simulink model "Cooling_System"  (R2019b)
settings: Solver=VariableStepAuto  StartTime=0.0  StopTime=3600  RelTol=1e-3
libraries: fl_lib x170, nesl_utility x49
(part 2 of 2)

== system Cooling_System/segment/Cell conductance23 ==
  Air-Iron Conductance : fl_lib/Thermal/Thermal Elements/Conductive Heat Transfer  area=0.014 m^2  thickness=2 mm  th_cond=0.0257 W/(m*K)  T_specify=off  T_priority=None  T=0 K  T_nominal_specify=off  T_nominal_unit=K  T_nominal_value=1  Q_specify=off  Q_priority=None  Q=0 W  Q_nominal_specify=off  Q_nominal_unit=W  Q_nominal_value=1
      settings: SourceProductName=Simscape
  Atmosphere Temperature : fl_lib/Thermal/Thermal Sources/Temperature Source  temperature=300 K
      settings: SourceProductName=Simscape
  Jules Power Losses : fl_lib/Thermal/Thermal Sources/Controlled Heat Flow Rate Source
      settings: SourceProductName=Simscape
  PS-Simulink Converter : nesl_utility/PS-Simulink Converter  PhysicalDomain=network_engine_domain  SubClassName=ps_output  LeftPortType=input  RightPortType=output  PseudoPeriodic=off  Frequencies=[]  Unit=1  AffineConversion=off
  Simulink-PS Converter : nesl_utility/Simulink-PS Converter  PhysicalDomain=network_engine_domain  SubClassName=ps_input  LeftPortType=input  RightPortType=output  PseudoPeriodic=off  Frequencies=[]  NoiseDistribution=none  NoiseParameters=[]  Unit=W  AffineConversion=off  FilteringAndDerivatives=zero  SimscapeFilterOrder=1  InputFilterTimeConstant=.001  UdotUserProvided=[]
  Stator Iron Thermal Mass : fl_lib/Thermal/Thermal Elements/Thermal Mass  mass=0.3 kg  sp_heat=460 J/kg/K  T_specify=off  T_priority=High  T=300 K  T_nominal_specify=off  T_nominal_unit=K  T_nominal_value=1  Q_specify=off  Q_priority=None  Q=0 W  Q_nominal_specify=off  Q_nominal_unit=W  Q_nominal_value=1
  Temperature Sensor : fl_lib/Thermal/Thermal Sensors/Temperature Sensor
  Thermal Reference : fl_lib/Thermal/Thermal Elements/Thermal Reference
  Thermal Resistance : fl_lib/Thermal/Thermal Elements/Thermal Resistance  resistance=1/(1.006*1.202*0.028*50.4/60*1000) K/W  T_specify=off  T_priority=None  T=0 K  T_nominal_specify=off  T_nominal_unit=K  T_nominal_value=1  Q_specify=off  Q_priority=None  Q=0 W  Q_nominal_specify=off  Q_nominal_unit=W  Q_nominal_value=1
      settings: SourceProductName=Simscape  SourceProductBaseCode=SS
  temp_Cell_A : PMIOPort  Side=Left
  temp_Cell_B : PMIOPort  Port=2  Side=Right
  tag scope: temp_cell_23=global
  wires:
  [Q_cell] -> Simulink-PS Converter/1
  PS-Simulink Converter/1 -> [temp_cell_23]
  connections:
  Jules Power Losses/LConn1 -- temp_Cell_A/RConn1 -- Temperature Sensor/RConn1 -- Stator Iron Thermal Mass/LConn1 -- Air-Iron Conductance/LConn1
  Air-Iron Conductance/RConn1 -- Thermal Resistance/LConn1 -- temp_Cell_B/RConn1 -- Temperature Sensor/LConn1
  Atmosphere Temperature/LConn1 -- Thermal Resistance/RConn1
  Jules Power Losses/RConn1 -- Simulink-PS Converter/RConn1
  PS-Simulink Converter/LConn1 -- Temperature Sensor/RConn2
  Thermal Reference/LConn1 -- Jules Power Losses/RConn2

== system Cooling_System/segment/Cell conductance24 ==
  Air-Iron Conductance : fl_lib/Thermal/Thermal Elements/Conductive Heat Transfer  area=0.014 m^2  thickness=2 mm  th_cond=0.0257 W/(m*K)  T_specify=off  T_priority=None  T=0 K  T_nominal_specify=off  T_nominal_unit=K  T_nominal_value=1  Q_specify=off  Q_priority=None  Q=0 W  Q_nominal_specify=off  Q_nominal_unit=W  Q_nominal_value=1
      settings: SourceProductName=Simscape
  Atmosphere Temperature : fl_lib/Thermal/Thermal Sources/Temperature Source  temperature=300 K
      settings: SourceProductName=Simscape
  Jules Power Losses : fl_lib/Thermal/Thermal Sources/Controlled Heat Flow Rate Source
      settings: SourceProductName=Simscape
  PS-Simulink Converter : nesl_utility/PS-Simulink Converter  PhysicalDomain=network_engine_domain  SubClassName=ps_output  LeftPortType=input  RightPortType=output  PseudoPeriodic=off  Frequencies=[]  Unit=1  AffineConversion=off
  Simulink-PS Converter : nesl_utility/Simulink-PS Converter  PhysicalDomain=network_engine_domain  SubClassName=ps_input  LeftPortType=input  RightPortType=output  PseudoPeriodic=off  Frequencies=[]  NoiseDistribution=none  NoiseParameters=[]  Unit=W  AffineConversion=off  FilteringAndDerivatives=zero  SimscapeFilterOrder=1  InputFilterTimeConstant=.001  UdotUserProvided=[]
  Stator Iron Thermal Mass : fl_lib/Thermal/Thermal Elements/Thermal Mass  mass=0.3 kg  sp_heat=460 J/kg/K  T_specify=off  T_priority=High  T=300 K  T_nominal_specify=off  T_nominal_unit=K  T_nominal_value=1  Q_specify=off  Q_priority=None  Q=0 W  Q_nominal_specify=off  Q_nominal_unit=W  Q_nominal_value=1
  Temperature Sensor : fl_lib/Thermal/Thermal Sensors/Temperature Sensor
  Thermal Reference : fl_lib/Thermal/Thermal Elements/Thermal Reference
  Thermal Resistance : fl_lib/Thermal/Thermal Elements/Thermal Resistance  resistance=1/(1.006*1.202*0.028*50.4/60*1000) K/W  T_specify=off  T_priority=None  T=0 K  T_nominal_specify=off  T_nominal_unit=K  T_nominal_value=1  Q_specify=off  Q_priority=None  Q=0 W  Q_nominal_specify=off  Q_nominal_unit=W  Q_nominal_value=1
      settings: SourceProductName=Simscape  SourceProductBaseCode=SS
  temp_Cell_A : PMIOPort  Side=Left
  temp_Cell_B : PMIOPort  Port=2  Side=Right
  tag scope: temp_cell_24=global
  wires:
  [Q_cell] -> Simulink-PS Converter/1
  PS-Simulink Converter/1 -> [temp_cell_24]
  connections:
  Jules Power Losses/LConn1 -- temp_Cell_A/RConn1 -- Temperature Sensor/RConn1 -- Stator Iron Thermal Mass/LConn1 -- Air-Iron Conductance/LConn1
  Air-Iron Conductance/RConn1 -- Thermal Resistance/LConn1 -- temp_Cell_B/RConn1 -- Temperature Sensor/LConn1
  Atmosphere Temperature/LConn1 -- Thermal Resistance/RConn1
  Jules Power Losses/RConn1 -- Simulink-PS Converter/RConn1
  PS-Simulink Converter/LConn1 -- Temperature Sensor/RConn2
  Thermal Reference/LConn1 -- Jules Power Losses/RConn2

== system Cooling_System/segment/Cell conductance3 ==
  Air-Iron Conductance : fl_lib/Thermal/Thermal Elements/Conductive Heat Transfer  area=0.014 m^2  thickness=2 mm  th_cond=0.0257 W/(m*K)  T_specify=off  T_priority=None  T=0 K  T_nominal_specify=off  T_nominal_unit=K  T_nominal_value=1  Q_specify=off  Q_priority=None  Q=0 W  Q_nominal_specify=off  Q_nominal_unit=W  Q_nominal_value=1
      settings: SourceProductName=Simscape
  Atmosphere Temperature : fl_lib/Thermal/Thermal Sources/Temperature Source  temperature=300 K
      settings: SourceProductName=Simscape
  Jules Power Losses : fl_lib/Thermal/Thermal Sources/Controlled Heat Flow Rate Source
      settings: SourceProductName=Simscape
  PS-Simulink Converter : nesl_utility/PS-Simulink Converter  PhysicalDomain=network_engine_domain  SubClassName=ps_output  LeftPortType=input  RightPortType=output  PseudoPeriodic=off  Frequencies=[]  Unit=1  AffineConversion=off
  Simulink-PS Converter : nesl_utility/Simulink-PS Converter  PhysicalDomain=network_engine_domain  SubClassName=ps_input  LeftPortType=input  RightPortType=output  PseudoPeriodic=off  Frequencies=[]  NoiseDistribution=none  NoiseParameters=[]  Unit=W  AffineConversion=off  FilteringAndDerivatives=zero  SimscapeFilterOrder=1  InputFilterTimeConstant=.001  UdotUserProvided=[]
  Stator Iron Thermal Mass : fl_lib/Thermal/Thermal Elements/Thermal Mass  mass=0.3 kg  sp_heat=460 J/kg/K  T_specify=off  T_priority=High  T=300 K  T_nominal_specify=off  T_nominal_unit=K  T_nominal_value=1  Q_specify=off  Q_priority=None  Q=0 W  Q_nominal_specify=off  Q_nominal_unit=W  Q_nominal_value=1
  Temperature Sensor : fl_lib/Thermal/Thermal Sensors/Temperature Sensor
  Thermal Reference : fl_lib/Thermal/Thermal Elements/Thermal Reference
  Thermal Resistance : fl_lib/Thermal/Thermal Elements/Thermal Resistance  resistance=1/(1.006*1.202*0.028*50.4/60*1000) K/W  T_specify=off  T_priority=None  T=0 K  T_nominal_specify=off  T_nominal_unit=K  T_nominal_value=1  Q_specify=off  Q_priority=None  Q=0 W  Q_nominal_specify=off  Q_nominal_unit=W  Q_nominal_value=1
      settings: SourceProductName=Simscape  SourceProductBaseCode=SS
  temp_Cell_A : PMIOPort  Side=Left
  temp_Cell_B : PMIOPort  Port=2  Side=Right
  tag scope: temp_cell_03=global
  wires:
  [Q_cell] -> Simulink-PS Converter/1
  PS-Simulink Converter/1 -> [temp_cell_03]
  connections:
  Jules Power Losses/LConn1 -- temp_Cell_A/RConn1 -- Temperature Sensor/RConn1 -- Stator Iron Thermal Mass/LConn1 -- Air-Iron Conductance/LConn1
  Air-Iron Conductance/RConn1 -- Thermal Resistance/LConn1 -- temp_Cell_B/RConn1 -- Temperature Sensor/LConn1
  Atmosphere Temperature/LConn1 -- Thermal Resistance/RConn1
  Jules Power Losses/RConn1 -- Simulink-PS Converter/RConn1
  PS-Simulink Converter/LConn1 -- Temperature Sensor/RConn2
  Thermal Reference/LConn1 -- Jules Power Losses/RConn2

== system Cooling_System/segment/Cell conductance4 ==
  Air-Iron Conductance : fl_lib/Thermal/Thermal Elements/Conductive Heat Transfer  area=0.014 m^2  thickness=2 mm  th_cond=0.0257 W/(m*K)  T_specify=off  T_priority=None  T=0 K  T_nominal_specify=off  T_nominal_unit=K  T_nominal_value=1  Q_specify=off  Q_priority=None  Q=0 W  Q_nominal_specify=off  Q_nominal_unit=W  Q_nominal_value=1
      settings: SourceProductName=Simscape
  Atmosphere Temperature : fl_lib/Thermal/Thermal Sources/Temperature Source  temperature=300 K
      settings: SourceProductName=Simscape
  Jules Power Losses : fl_lib/Thermal/Thermal Sources/Controlled Heat Flow Rate Source
      settings: SourceProductName=Simscape
  PS-Simulink Converter : nesl_utility/PS-Simulink Converter  PhysicalDomain=network_engine_domain  SubClassName=ps_output  LeftPortType=input  RightPortType=output  PseudoPeriodic=off  Frequencies=[]  Unit=1  AffineConversion=off
  Simulink-PS Converter : nesl_utility/Simulink-PS Converter  PhysicalDomain=network_engine_domain  SubClassName=ps_input  LeftPortType=input  RightPortType=output  PseudoPeriodic=off  Frequencies=[]  NoiseDistribution=none  NoiseParameters=[]  Unit=W  AffineConversion=off  FilteringAndDerivatives=zero  SimscapeFilterOrder=1  InputFilterTimeConstant=.001  UdotUserProvided=[]
  Stator Iron Thermal Mass : fl_lib/Thermal/Thermal Elements/Thermal Mass  mass=0.3 kg  sp_heat=460 J/kg/K  T_specify=off  T_priority=High  T=300 K  T_nominal_specify=off  T_nominal_unit=K  T_nominal_value=1  Q_specify=off  Q_priority=None  Q=0 W  Q_nominal_specify=off  Q_nominal_unit=W  Q_nominal_value=1
  Temperature Sensor : fl_lib/Thermal/Thermal Sensors/Temperature Sensor
  Thermal Reference : fl_lib/Thermal/Thermal Elements/Thermal Reference
  Thermal Resistance : fl_lib/Thermal/Thermal Elements/Thermal Resistance  resistance=1/(1.006*1.202*0.028*50.4/60*1000) K/W  T_specify=off  T_priority=None  T=0 K  T_nominal_specify=off  T_nominal_unit=K  T_nominal_value=1  Q_specify=off  Q_priority=None  Q=0 W  Q_nominal_specify=off  Q_nominal_unit=W  Q_nominal_value=1
      settings: SourceProductName=Simscape  SourceProductBaseCode=SS
  temp_Cell_A : PMIOPort  Side=Left
  temp_Cell_B : PMIOPort  Port=2  Side=Right
  tag scope: temp_cell_04=global
  wires:
  [Q_cell] -> Simulink-PS Converter/1
  PS-Simulink Converter/1 -> [temp_cell_04]
  connections:
  Jules Power Losses/LConn1 -- temp_Cell_A/RConn1 -- Temperature Sensor/RConn1 -- Stator Iron Thermal Mass/LConn1 -- Air-Iron Conductance/LConn1
  Air-Iron Conductance/RConn1 -- Thermal Resistance/LConn1 -- temp_Cell_B/RConn1 -- Temperature Sensor/LConn1
  Atmosphere Temperature/LConn1 -- Thermal Resistance/RConn1
  Jules Power Losses/RConn1 -- Simulink-PS Converter/RConn1
  PS-Simulink Converter/LConn1 -- Temperature Sensor/RConn2
  Thermal Reference/LConn1 -- Jules Power Losses/RConn2

== system Cooling_System/segment/Cell conductance5 ==
  Air-Iron Conductance : fl_lib/Thermal/Thermal Elements/Conductive Heat Transfer  area=0.014 m^2  thickness=2 mm  th_cond=0.0257 W/(m*K)  T_specify=off  T_priority=None  T=0 K  T_nominal_specify=off  T_nominal_unit=K  T_nominal_value=1  Q_specify=off  Q_priority=None  Q=0 W  Q_nominal_specify=off  Q_nominal_unit=W  Q_nominal_value=1
      settings: SourceProductName=Simscape
  Atmosphere Temperature : fl_lib/Thermal/Thermal Sources/Temperature Source  temperature=300 K
      settings: SourceProductName=Simscape
  Jules Power Losses : fl_lib/Thermal/Thermal Sources/Controlled Heat Flow Rate Source
      settings: SourceProductName=Simscape
  PS-Simulink Converter : nesl_utility/PS-Simulink Converter  PhysicalDomain=network_engine_domain  SubClassName=ps_output  LeftPortType=input  RightPortType=output  PseudoPeriodic=off  Frequencies=[]  Unit=1  AffineConversion=off
  Simulink-PS Converter : nesl_utility/Simulink-PS Converter  PhysicalDomain=network_engine_domain  SubClassName=ps_input  LeftPortType=input  RightPortType=output  PseudoPeriodic=off  Frequencies=[]  NoiseDistribution=none  NoiseParameters=[]  Unit=W  AffineConversion=off  FilteringAndDerivatives=zero  SimscapeFilterOrder=1  InputFilterTimeConstant=.001  UdotUserProvided=[]
  Stator Iron Thermal Mass : fl_lib/Thermal/Thermal Elements/Thermal Mass  mass=0.3 kg  sp_heat=460 J/kg/K  T_specify=off  T_priority=High  T=300 K  T_nominal_specify=off  T_nominal_unit=K  T_nominal_value=1  Q_specify=off  Q_priority=None  Q=0 W  Q_nominal_specify=off  Q_nominal_unit=W  Q_nominal_value=1
  Temperature Sensor : fl_lib/Thermal/Thermal Sensors/Temperature Sensor
  Thermal Reference : fl_lib/Thermal/Thermal Elements/Thermal Reference
  Thermal Resistance : fl_lib/Thermal/Thermal Elements/Thermal Resistance  resistance=1/(1.006*1.202*0.028*50.4/60*1000) K/W  T_specify=off  T_priority=None  T=0 K  T_nominal_specify=off  T_nominal_unit=K  T_nominal_value=1  Q_specify=off  Q_priority=None  Q=0 W  Q_nominal_specify=off  Q_nominal_unit=W  Q_nominal_value=1
      settings: SourceProductName=Simscape  SourceProductBaseCode=SS
  temp_Cell_A : PMIOPort  Side=Left
  temp_Cell_B : PMIOPort  Port=2  Side=Right
  tag scope: temp_cell_05=global
  wires:
  [Q_cell] -> Simulink-PS Converter/1
  PS-Simulink Converter/1 -> [temp_cell_05]
  connections:
  Jules Power Losses/LConn1 -- temp_Cell_A/RConn1 -- Temperature Sensor/RConn1 -- Stator Iron Thermal Mass/LConn1 -- Air-Iron Conductance/LConn1
  Air-Iron Conductance/RConn1 -- Thermal Resistance/LConn1 -- temp_Cell_B/RConn1 -- Temperature Sensor/LConn1
  Atmosphere Temperature/LConn1 -- Thermal Resistance/RConn1
  Jules Power Losses/RConn1 -- Simulink-PS Converter/RConn1
  PS-Simulink Converter/LConn1 -- Temperature Sensor/RConn2
  Thermal Reference/LConn1 -- Jules Power Losses/RConn2

== system Cooling_System/segment/Cell conductance6 ==
  Air-Iron Conductance : fl_lib/Thermal/Thermal Elements/Conductive Heat Transfer  area=0.014 m^2  thickness=2 mm  th_cond=0.0257 W/(m*K)  T_specify=off  T_priority=None  T=0 K  T_nominal_specify=off  T_nominal_unit=K  T_nominal_value=1  Q_specify=off  Q_priority=None  Q=0 W  Q_nominal_specify=off  Q_nominal_unit=W  Q_nominal_value=1
      settings: SourceProductName=Simscape
  Atmosphere Temperature : fl_lib/Thermal/Thermal Sources/Temperature Source  temperature=300 K
      settings: SourceProductName=Simscape
  Jules Power Losses : fl_lib/Thermal/Thermal Sources/Controlled Heat Flow Rate Source
      settings: SourceProductName=Simscape
  PS-Simulink Converter : nesl_utility/PS-Simulink Converter  PhysicalDomain=network_engine_domain  SubClassName=ps_output  LeftPortType=input  RightPortType=output  PseudoPeriodic=off  Frequencies=[]  Unit=1  AffineConversion=off
  Simulink-PS Converter : nesl_utility/Simulink-PS Converter  PhysicalDomain=network_engine_domain  SubClassName=ps_input  LeftPortType=input  RightPortType=output  PseudoPeriodic=off  Frequencies=[]  NoiseDistribution=none  NoiseParameters=[]  Unit=W  AffineConversion=off  FilteringAndDerivatives=zero  SimscapeFilterOrder=1  InputFilterTimeConstant=.001  UdotUserProvided=[]
  Stator Iron Thermal Mass : fl_lib/Thermal/Thermal Elements/Thermal Mass  mass=0.3 kg  sp_heat=460 J/kg/K  T_specify=off  T_priority=High  T=300 K  T_nominal_specify=off  T_nominal_unit=K  T_nominal_value=1  Q_specify=off  Q_priority=None  Q=0 W  Q_nominal_specify=off  Q_nominal_unit=W  Q_nominal_value=1
  Temperature Sensor : fl_lib/Thermal/Thermal Sensors/Temperature Sensor
  Thermal Reference : fl_lib/Thermal/Thermal Elements/Thermal Reference
  Thermal Resistance : fl_lib/Thermal/Thermal Elements/Thermal Resistance  resistance=1/(1.006*1.202*0.028*50.4/60*1000) K/W  T_specify=off  T_priority=None  T=0 K  T_nominal_specify=off  T_nominal_unit=K  T_nominal_value=1  Q_specify=off  Q_priority=None  Q=0 W  Q_nominal_specify=off  Q_nominal_unit=W  Q_nominal_value=1
      settings: SourceProductName=Simscape  SourceProductBaseCode=SS
  temp_Cell_A : PMIOPort  Side=Left
  temp_Cell_B : PMIOPort  Port=2  Side=Right
  tag scope: temp_cell_06=global
  wires:
  [Q_cell] -> Simulink-PS Converter/1
  PS-Simulink Converter/1 -> [temp_cell_06]
  connections:
  Jules Power Losses/LConn1 -- temp_Cell_A/RConn1 -- Temperature Sensor/RConn1 -- Stator Iron Thermal Mass/LConn1 -- Air-Iron Conductance/LConn1
  Air-Iron Conductance/RConn1 -- Thermal Resistance/LConn1 -- temp_Cell_B/RConn1 -- Temperature Sensor/LConn1
  Atmosphere Temperature/LConn1 -- Thermal Resistance/RConn1
  Jules Power Losses/RConn1 -- Simulink-PS Converter/RConn1
  PS-Simulink Converter/LConn1 -- Temperature Sensor/RConn2
  Thermal Reference/LConn1 -- Jules Power Losses/RConn2

== system Cooling_System/segment/Cell conductance7 ==
  Air-Iron Conductance : fl_lib/Thermal/Thermal Elements/Conductive Heat Transfer  area=0.014 m^2  thickness=2 mm  th_cond=0.0257 W/(m*K)  T_specify=off  T_priority=None  T=0 K  T_nominal_specify=off  T_nominal_unit=K  T_nominal_value=1  Q_specify=off  Q_priority=None  Q=0 W  Q_nominal_specify=off  Q_nominal_unit=W  Q_nominal_value=1
      settings: SourceProductName=Simscape
  Atmosphere Temperature : fl_lib/Thermal/Thermal Sources/Temperature Source  temperature=300 K
      settings: SourceProductName=Simscape
  Jules Power Losses : fl_lib/Thermal/Thermal Sources/Controlled Heat Flow Rate Source
      settings: SourceProductName=Simscape
  PS-Simulink Converter : nesl_utility/PS-Simulink Converter  PhysicalDomain=network_engine_domain  SubClassName=ps_output  LeftPortType=input  RightPortType=output  PseudoPeriodic=off  Frequencies=[]  Unit=1  AffineConversion=off
  Simulink-PS Converter : nesl_utility/Simulink-PS Converter  PhysicalDomain=network_engine_domain  SubClassName=ps_input  LeftPortType=input  RightPortType=output  PseudoPeriodic=off  Frequencies=[]  NoiseDistribution=none  NoiseParameters=[]  Unit=W  AffineConversion=off  FilteringAndDerivatives=zero  SimscapeFilterOrder=1  InputFilterTimeConstant=.001  UdotUserProvided=[]
  Stator Iron Thermal Mass : fl_lib/Thermal/Thermal Elements/Thermal Mass  mass=0.3 kg  sp_heat=460 J/kg/K  T_specify=off  T_priority=High  T=300 K  T_nominal_specify=off  T_nominal_unit=K  T_nominal_value=1  Q_specify=off  Q_priority=None  Q=0 W  Q_nominal_specify=off  Q_nominal_unit=W  Q_nominal_value=1
  Temperature Sensor : fl_lib/Thermal/Thermal Sensors/Temperature Sensor
  Thermal Reference : fl_lib/Thermal/Thermal Elements/Thermal Reference
  Thermal Resistance : fl_lib/Thermal/Thermal Elements/Thermal Resistance  resistance=1/(1.006*1.202*0.028*50.4/60*1000) K/W  T_specify=off  T_priority=None  T=0 K  T_nominal_specify=off  T_nominal_unit=K  T_nominal_value=1  Q_specify=off  Q_priority=None  Q=0 W  Q_nominal_specify=off  Q_nominal_unit=W  Q_nominal_value=1
      settings: SourceProductName=Simscape  SourceProductBaseCode=SS
  temp_Cell_A : PMIOPort  Side=Left
  temp_Cell_B : PMIOPort  Port=2  Side=Right
  tag scope: temp_cell_07=global
  wires:
  [Q_cell] -> Simulink-PS Converter/1
  PS-Simulink Converter/1 -> [temp_cell_07]
  connections:
  Jules Power Losses/LConn1 -- temp_Cell_A/RConn1 -- Temperature Sensor/RConn1 -- Stator Iron Thermal Mass/LConn1 -- Air-Iron Conductance/LConn1
  Air-Iron Conductance/RConn1 -- Thermal Resistance/LConn1 -- temp_Cell_B/RConn1 -- Temperature Sensor/LConn1
  Atmosphere Temperature/LConn1 -- Thermal Resistance/RConn1
  Jules Power Losses/RConn1 -- Simulink-PS Converter/RConn1
  PS-Simulink Converter/LConn1 -- Temperature Sensor/RConn2
  Thermal Reference/LConn1 -- Jules Power Losses/RConn2

== system Cooling_System/segment/Cell conductance8 ==
  Air-Iron Conductance : fl_lib/Thermal/Thermal Elements/Conductive Heat Transfer  area=0.014 m^2  thickness=2 mm  th_cond=0.0257 W/(m*K)  T_specify=off  T_priority=None  T=0 K  T_nominal_specify=off  T_nominal_unit=K  T_nominal_value=1  Q_specify=off  Q_priority=None  Q=0 W  Q_nominal_specify=off  Q_nominal_unit=W  Q_nominal_value=1
      settings: SourceProductName=Simscape
  Atmosphere Temperature : fl_lib/Thermal/Thermal Sources/Temperature Source  temperature=300 K
      settings: SourceProductName=Simscape
  Jules Power Losses : fl_lib/Thermal/Thermal Sources/Controlled Heat Flow Rate Source
      settings: SourceProductName=Simscape
  PS-Simulink Converter : nesl_utility/PS-Simulink Converter  PhysicalDomain=network_engine_domain  SubClassName=ps_output  LeftPortType=input  RightPortType=output  PseudoPeriodic=off  Frequencies=[]  Unit=1  AffineConversion=off
  Simulink-PS Converter : nesl_utility/Simulink-PS Converter  PhysicalDomain=network_engine_domain  SubClassName=ps_input  LeftPortType=input  RightPortType=output  PseudoPeriodic=off  Frequencies=[]  NoiseDistribution=none  NoiseParameters=[]  Unit=W  AffineConversion=off  FilteringAndDerivatives=zero  SimscapeFilterOrder=1  InputFilterTimeConstant=.001  UdotUserProvided=[]
  Stator Iron Thermal Mass : fl_lib/Thermal/Thermal Elements/Thermal Mass  mass=0.3 kg  sp_heat=460 J/kg/K  T_specify=off  T_priority=High  T=300 K  T_nominal_specify=off  T_nominal_unit=K  T_nominal_value=1  Q_specify=off  Q_priority=None  Q=0 W  Q_nominal_specify=off  Q_nominal_unit=W  Q_nominal_value=1
  Temperature Sensor : fl_lib/Thermal/Thermal Sensors/Temperature Sensor
  Thermal Reference : fl_lib/Thermal/Thermal Elements/Thermal Reference
  Thermal Resistance : fl_lib/Thermal/Thermal Elements/Thermal Resistance  resistance=1/(1.006*1.202*0.028*50.4/60*1000) K/W  T_specify=off  T_priority=None  T=0 K  T_nominal_specify=off  T_nominal_unit=K  T_nominal_value=1  Q_specify=off  Q_priority=None  Q=0 W  Q_nominal_specify=off  Q_nominal_unit=W  Q_nominal_value=1
      settings: SourceProductName=Simscape  SourceProductBaseCode=SS
  temp_Cell_A : PMIOPort  Side=Left
  temp_Cell_B : PMIOPort  Port=2  Side=Right
  tag scope: temp_cell_08=global
  wires:
  [Q_cell] -> Simulink-PS Converter/1
  PS-Simulink Converter/1 -> [temp_cell_08]
  connections:
  Jules Power Losses/LConn1 -- temp_Cell_A/RConn1 -- Temperature Sensor/RConn1 -- Stator Iron Thermal Mass/LConn1 -- Air-Iron Conductance/LConn1
  Air-Iron Conductance/RConn1 -- Thermal Resistance/LConn1 -- temp_Cell_B/RConn1 -- Temperature Sensor/LConn1
  Atmosphere Temperature/LConn1 -- Thermal Resistance/RConn1
  Jules Power Losses/RConn1 -- Simulink-PS Converter/RConn1
  PS-Simulink Converter/LConn1 -- Temperature Sensor/RConn2
  Thermal Reference/LConn1 -- Jules Power Losses/RConn2

== system Cooling_System/segment/Cell conductance9 ==
  Air-Iron Conductance : fl_lib/Thermal/Thermal Elements/Conductive Heat Transfer  area=0.014 m^2  thickness=2 mm  th_cond=0.0257 W/(m*K)  T_specify=off  T_priority=None  T=0 K  T_nominal_specify=off  T_nominal_unit=K  T_nominal_value=1  Q_specify=off  Q_priority=None  Q=0 W  Q_nominal_specify=off  Q_nominal_unit=W  Q_nominal_value=1
      settings: SourceProductName=Simscape
  Atmosphere Temperature : fl_lib/Thermal/Thermal Sources/Temperature Source  temperature=300 K
      settings: SourceProductName=Simscape
  Jules Power Losses : fl_lib/Thermal/Thermal Sources/Controlled Heat Flow Rate Source
      settings: SourceProductName=Simscape
  PS-Simulink Converter : nesl_utility/PS-Simulink Converter  PhysicalDomain=network_engine_domain  SubClassName=ps_output  LeftPortType=input  RightPortType=output  PseudoPeriodic=off  Frequencies=[]  Unit=1  AffineConversion=off
  Simulink-PS Converter : nesl_utility/Simulink-PS Converter  PhysicalDomain=network_engine_domain  SubClassName=ps_input  LeftPortType=input  RightPortType=output  PseudoPeriodic=off  Frequencies=[]  NoiseDistribution=none  NoiseParameters=[]  Unit=W  AffineConversion=off  FilteringAndDerivatives=zero  SimscapeFilterOrder=1  InputFilterTimeConstant=.001  UdotUserProvided=[]
  Stator Iron Thermal Mass : fl_lib/Thermal/Thermal Elements/Thermal Mass  mass=0.3 kg  sp_heat=460 J/kg/K  T_specify=off  T_priority=High  T=300 K  T_nominal_specify=off  T_nominal_unit=K  T_nominal_value=1  Q_specify=off  Q_priority=None  Q=0 W  Q_nominal_specify=off  Q_nominal_unit=W  Q_nominal_value=1
  Temperature Sensor : fl_lib/Thermal/Thermal Sensors/Temperature Sensor
  Thermal Reference : fl_lib/Thermal/Thermal Elements/Thermal Reference
  Thermal Resistance : fl_lib/Thermal/Thermal Elements/Thermal Resistance  resistance=1/(1.006*1.202*0.028*50.4/60*1000) K/W  T_specify=off  T_priority=None  T=0 K  T_nominal_specify=off  T_nominal_unit=K  T_nominal_value=1  Q_specify=off  Q_priority=None  Q=0 W  Q_nominal_specify=off  Q_nominal_unit=W  Q_nominal_value=1
      settings: SourceProductName=Simscape  SourceProductBaseCode=SS
  temp_Cell_A : PMIOPort  Side=Left
  temp_Cell_B : PMIOPort  Port=2  Side=Right
  tag scope: temp_cell_09=global
  wires:
  [Q_cell] -> Simulink-PS Converter/1
  PS-Simulink Converter/1 -> [temp_cell_09]
  connections:
  Jules Power Losses/LConn1 -- temp_Cell_A/RConn1 -- Temperature Sensor/RConn1 -- Stator Iron Thermal Mass/LConn1 -- Air-Iron Conductance/LConn1
  Air-Iron Conductance/RConn1 -- Thermal Resistance/LConn1 -- temp_Cell_B/RConn1 -- Temperature Sensor/LConn1
  Atmosphere Temperature/LConn1 -- Thermal Resistance/RConn1
  Jules Power Losses/RConn1 -- Simulink-PS Converter/RConn1
  PS-Simulink Converter/LConn1 -- Temperature Sensor/RConn2
  Thermal Reference/LConn1 -- Jules Power Losses/RConn2

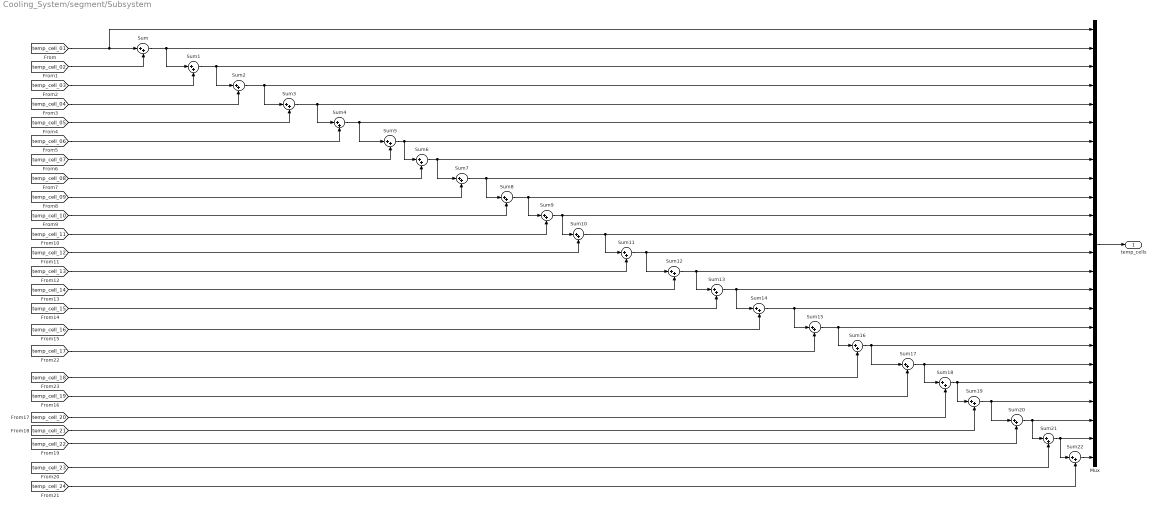
== system Cooling_System/segment/Subsystem ==
  Mux : Mux  Inputs=24
  Sum{,1..22} (23 alike) : Sum  Inputs=|++
  temp_cells : Outport
  wires:
  [temp_cell_13] -> Sum11/2
  Sum12/1 -> Sum13/1, Mux/14
  [temp_cell_14] -> Sum12/2
  [temp_cell_09] -> Sum7/2
  [temp_cell_10] -> Sum8/2
  Sum1/1 -> Mux/3, Sum2/1
  [temp_cell_11] -> Sum9/2
  [temp_cell_12] -> Sum10/2
  [temp_cell_07] -> Sum5/2
  [temp_cell_08] -> Sum6/2
  [temp_cell_06] -> Sum4/2
  [temp_cell_05] -> Sum3/2
  [temp_cell_04] -> Sum2/2
  Sum10/1 -> Mux/12, Sum11/1
  Mux/1 -> temp_cells/1
  Sum11/1 -> Mux/13, Sum12/1
  [temp_cell_02] -> Sum/2
  [temp_cell_03] -> Sum1/2
  Sum9/1 -> Mux/11, Sum10/1
  Sum8/1 -> Mux/10, Sum9/1
  Sum4/1 -> Mux/6, Sum5/1
  Sum7/1 -> Mux/9, Sum8/1
  Sum5/1 -> Mux/7, Sum6/1
  Sum6/1 -> Sum7/1, Mux/8
  Sum3/1 -> Mux/5, Sum4/1
  Sum2/1 -> Mux/4, Sum3/1
  [temp_cell_01] -> Mux/1, Sum/1
  Sum/1 -> Sum1/1, Mux/2
  [temp_cell_15] -> Sum13/2
  Sum13/1 -> Sum14/1, Mux/15
  Sum14/1 -> Sum15/1, Mux/16
  [temp_cell_16] -> Sum14/2
  Sum15/1 -> Sum16/1, Mux/17
  [temp_cell_17] -> Sum15/2
  Sum16/1 -> Mux/18, Sum17/1
  [temp_cell_18] -> Sum16/2
  Sum17/1 -> Sum18/1, Mux/19
  [temp_cell_19] -> Sum17/2
  Sum18/1 -> Sum19/1, Mux/20
  [temp_cell_20] -> Sum18/2
  Sum19/1 -> Sum20/1, Mux/21
  [temp_cell_21] -> Sum19/2
  Sum20/1 -> Sum21/1, Mux/22
  [temp_cell_22] -> Sum20/2
  Sum21/1 -> Sum22/1, Mux/23
  [temp_cell_23] -> Sum21/2
  Sum22/1 -> Mux/24
  [temp_cell_24] -> Sum22/2
